simulink model "reverse"  (R2021a)
settings: Solver=VariableStepAuto  StartTime=0.0  StopTime=10.0  RelTol=1e-3
settings Model: Creator=abdul  LastModifiedBy=abdul

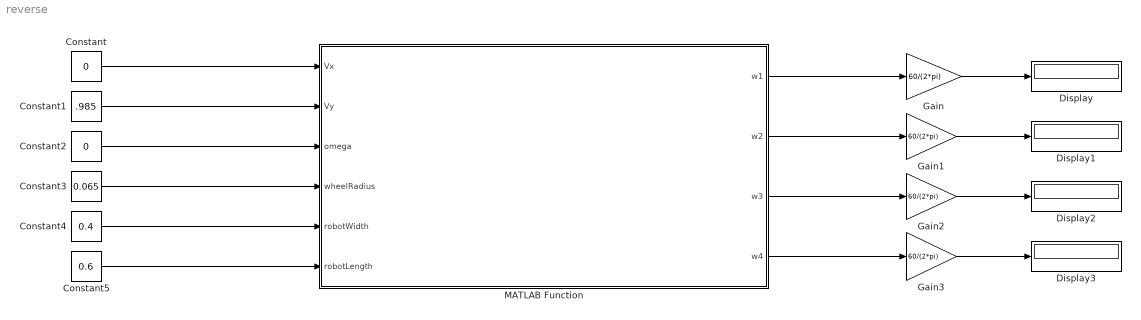
== system reverse ==
  Constant : Constant  Value=0
  Constant1 : Constant  Value=.985
  Constant2 : Constant  Value=0
  Constant3 : Constant  Value=0.065
  Constant4 : Constant  Value=0.4
  Constant5 : Constant  Value=0.6
  Display{,1..3} (4 alike) : Display
  Gain{,1..3} (4 alike) : Gain  Gain=60/(2*pi)
  MATLAB Function : MATLAB Function  TreatAsAtomicUnit=on
  wires:
  Constant/1 -> MATLAB Function/1(Vx)
  Constant1/1 -> MATLAB Function/2(Vy)
  Constant2/1 -> MATLAB Function/3(omega)
  Constant3/1 -> MATLAB Function/4(wheelRadius)
  Constant4/1 -> MATLAB Function/5(robotWidth)
  Constant5/1 -> MATLAB Function/6(robotLength)
  MATLAB Function/1(w1) -> Gain/1
  MATLAB Function/2(w2) -> Gain1/1
  MATLAB Function/3(w3) -> Gain2/1
  MATLAB Function/4(w4) -> Gain3/1
  Gain/1 -> Display/1
  Gain1/1 -> Display1/1
  Gain2/1 -> Display2/1
  Gain3/1 -> Display3/1

== matlab function reverse/MATLAB Function ==
  data: Vx input; w1 output; Vy input; omega input; wheelRadius input; robotWidth input; robotLength input; w2 output; w3 output; w4 output
function [w1, w2, w3, w4] = mecanumReverseKinematics(Vx, Vy, omega, wheelRadius, robotWidth, robotLength)
    % Reverse Kinematics for Mecanum Wheeled Robot
    R = wheelRadius;
    L = robotWidth / 2;
    d = robotLength / 2;
    o=L+d;

    M = [
         1   ,-1  ,-o ;
         1   ,1   , o ;
         1   ,1   ,-o ;
         1   ,-1  ,-o ;
        
    ];

    X_dot = [Vx ; Vy ; omega];
    W = 1/R.*M * X_dot;

    w1 = W(1);
    w2 = W(2);
    w3 = W(3);
    w4 = W(4);
end
